simulink model "test_model"  (R2024a)
settings: Solver=VariableStepAuto  StartTime=0.0  StopTime=10.0  RelTol=1e-3
undefined symbols (not defined in the file): DiscIntNeverNeededParam
settings Model: Creator=jeonghyun  LastModifiedBy=gluts

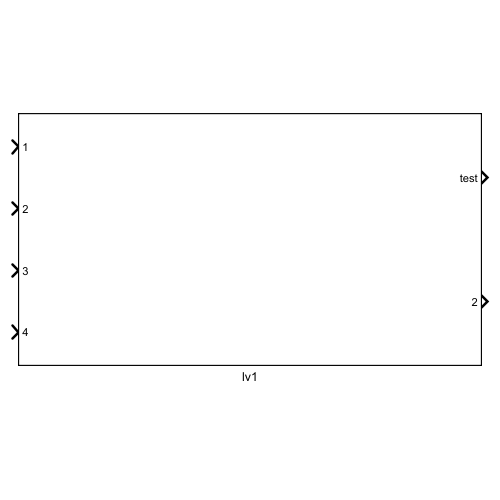
[thumbnail: Simulink's stored preview of the top-level diagram]
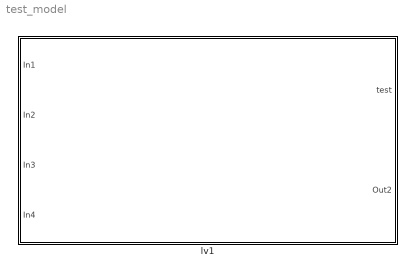
== system test_model ==
  lv1 : Subsystem

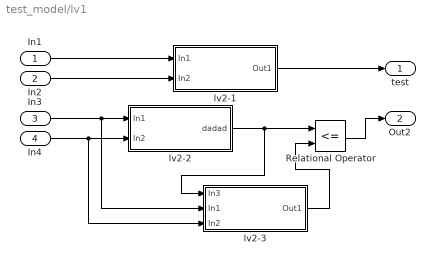
== system test_model/lv1 ==
  In1 : Inport
  In2 : Inport  Port=2
  In3 : Inport  Port=3
  In4 : Inport  Port=4
  Relational Operator : RelationalOperator  Operator=<=  OutDataTypeStr=boolean  RndMeth=Simplest  InputSameDT=off
  lv2-1 : Subsystem  TreatAsAtomicUnit=on
  lv2-2 : Subsystem
  lv2-3 : Subsystem
  test : Outport  LockScale=on
  Out2 : Outport  Port=2
  wires:
  In1/1 -> lv2-1/1(In1)
  In2/1 -> lv2-1/2(In2)
  In3/1 -> lv2-3/2(In1), lv2-2/1(In1)
  In4/1 -> lv2-3/3(In2), lv2-2/2(In2)
  lv2-1/1(Out1) -> test/1
  lv2-3/1(Out1) -> Relational Operator/2
  Relational Operator/1 -> Out2/1
  lv2-2/1(dadad) -> Relational Operator/1, lv2-3/1(In3)

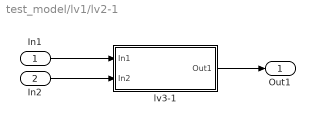
== system test_model/lv1/lv2-1 ==
  In1 : Inport  LockScale=on
  In2 : Inport  Port=2  LockScale=on
  lv3-1 : Subsystem
  Out1 : Outport  LockScale=on
  wires:
  In1/1 -> lv3-1/1(In1)
  In2/1 -> lv3-1/2(In2)
  lv3-1/1(Out1) -> Out1/1

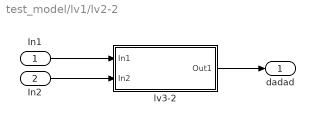
== system test_model/lv1/lv2-2 ==
  In1 : Inport
  In2 : Inport  Port=2
  lv3-2 : Subsystem
  dadad : Outport
  wires:
  In1/1 -> lv3-2/1(In1)
  In2/1 -> lv3-2/2(In2)
  lv3-2/1(Out1) -> dadad/1

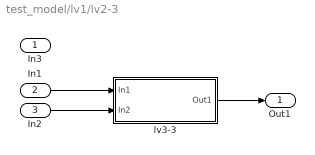
== system test_model/lv1/lv2-3 ==
  In3 : Inport
  In1 : Inport  Port=2
  In2 : Inport  Port=3
  lv3-3 : Subsystem
  Out1 : Outport
  wires:
  In1/1 -> lv3-3/1(In1)
  In2/1 -> lv3-3/2(In2)
  lv3-3/1(Out1) -> Out1/1

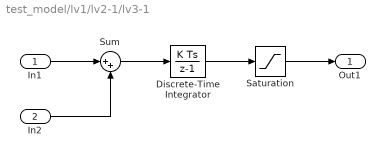
== system test_model/lv1/lv2-1/lv3-1 ==
  In1 : Inport
  In2 : Inport  Port=2
  Discrete-Time Integrator : DiscreteIntegrator  SampleTime=-1  ICPrevOutput=DiscIntNeverNeededParam  ICPrevScaledInput=DiscIntNeverNeededParam
  Saturation : Saturate
  Sum : Sum  Inputs=|++
  Out1 : Outport
  wires:
  In1/1 -> Sum/1
  In2/1 -> Sum/2
  Sum/1 -> Discrete-Time Integrator/1
  Discrete-Time Integrator/1 -> Saturation/1
  Saturation/1 -> Out1/1

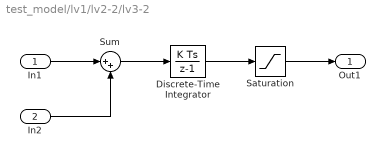
== system test_model/lv1/lv2-2/lv3-2 ==
  In1 : Inport
  In2 : Inport  Port=2
  Discrete-Time Integrator : DiscreteIntegrator  SampleTime=-1  ICPrevOutput=DiscIntNeverNeededParam  ICPrevScaledInput=DiscIntNeverNeededParam
  Saturation : Saturate
  Sum : Sum  Inputs=|++
  Out1 : Outport
  wires:
  In1/1 -> Sum/1
  In2/1 -> Sum/2
  Sum/1 -> Discrete-Time Integrator/1
  Discrete-Time Integrator/1 -> Saturation/1
  Saturation/1 -> Out1/1

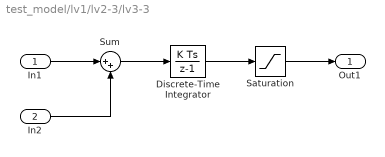
== system test_model/lv1/lv2-3/lv3-3 ==
  In1 : Inport
  In2 : Inport  Port=2
  Discrete-Time Integrator : DiscreteIntegrator  SampleTime=-1  ICPrevOutput=DiscIntNeverNeededParam  ICPrevScaledInput=DiscIntNeverNeededParam
  Saturation : Saturate
  Sum : Sum  Inputs=|++
  Out1 : Outport
  wires:
  In1/1 -> Sum/1
  In2/1 -> Sum/2
  Sum/1 -> Discrete-Time Integrator/1
  Discrete-Time Integrator/1 -> Saturation/1
  Saturation/1 -> Out1/1
